simulink model "FinalProject_EE547_Step15"  (R2018b)
settings: Solver=VariableStepAuto  StartTime=0.0  StopTime=10.0  RelTol=1e-3
values from neighbouring files (symbols this model uses):
  C = eye(4)    [Goniodsky_Mistry_EE547_ProjectCode.m]
  D = zeros(4,1)    [Goniodsky_Mistry_EE547_ProjectCode.m]
  K = place(A,B,poles1)    [Goniodsky_Mistry_EE547_ProjectCode.m]
  L = L'    [Goniodsky_Mistry_EE547_ProjectCode.m]
  xhatini = [0;0;0;0]    [Goniodsky_Mistry_EE547_ProjectCode.m]
undefined symbols (not defined in the file or in its folder): A, B
settings Model: Creator=GAJJAR  LastModifiedBy=GAJJAR

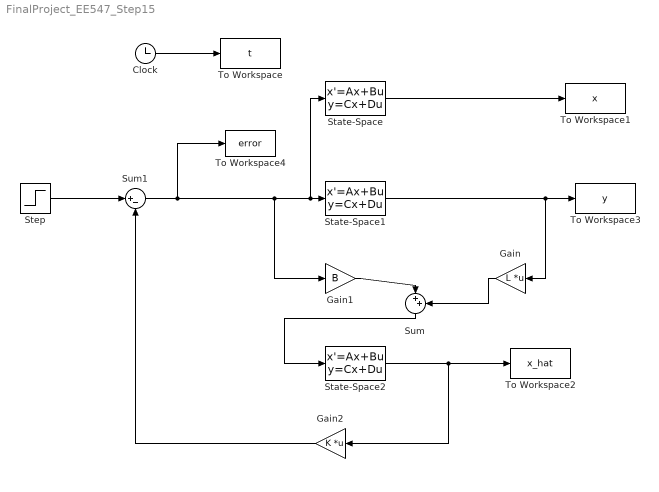
== system FinalProject_EE547_Step15 ==
  Clock : Clock
  Gain : Gain  Gain=L  Multiplication=Matrix(K*u)
  Gain1 : Gain  Gain=B
  Gain2 : Gain  Gain=K  Multiplication=Matrix(K*u)
  State-Space : StateSpace  A=A  B=B  C=eye(4)  D=zeros(4,1)  InitialCondition=0
  State-Space1 : StateSpace  A=A  B=B  C=C  D=D  InitialCondition=0
  State-Space2 : StateSpace  A=A-L*C  B=eye(4)  C=eye(4)  D=zeros(4,4)  InitialCondition=xhatini
  Step : Step  Time=0  SampleTime=0
  Sum : Sum  Inputs=|++
  Sum1 : Sum  Inputs=|+-
  To Workspace : ToWorkspace  VariableName=t  SampleTime=-1
  To Workspace1 : ToWorkspace  VariableName=x  SampleTime=-1
  To Workspace2 : ToWorkspace  VariableName=x_hat  SampleTime=-1
  To Workspace3 : ToWorkspace  VariableName=y  SampleTime=-1
  To Workspace4 : ToWorkspace  VariableName=error  SampleTime=-1
      settings: Save2DSignal=2-D array (concatenate along first dimension)
  wires:
  Gain1/1 -> Sum/1
  Sum/1 -> State-Space2/1
  Gain/1 -> Sum/2
  State-Space1/1 -> Gain/1, To Workspace3/1
  State-Space2/1 -> Gain2/1, To Workspace2/1
  Clock/1 -> To Workspace/1
  State-Space/1 -> To Workspace1/1
  Step/1 -> Sum1/1
  Sum1/1 -> To Workspace4/1, Gain1/1, State-Space/1, State-Space1/1
  Gain2/1 -> Sum1/2
